simulink subsystem "Regler"  (R2021b)
settings: Solver=VariableStepAuto  StartTime=0.0  StopTime=10.0  RelTol=1e-3
undefined symbols (not defined in the file or in its folder): SimParam
settings Model: Creator=tim  LastModifiedBy=tim

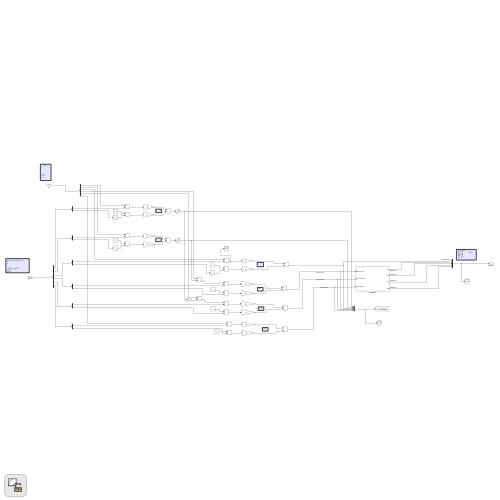
[thumbnail: Simulink's stored preview of the top-level diagram]
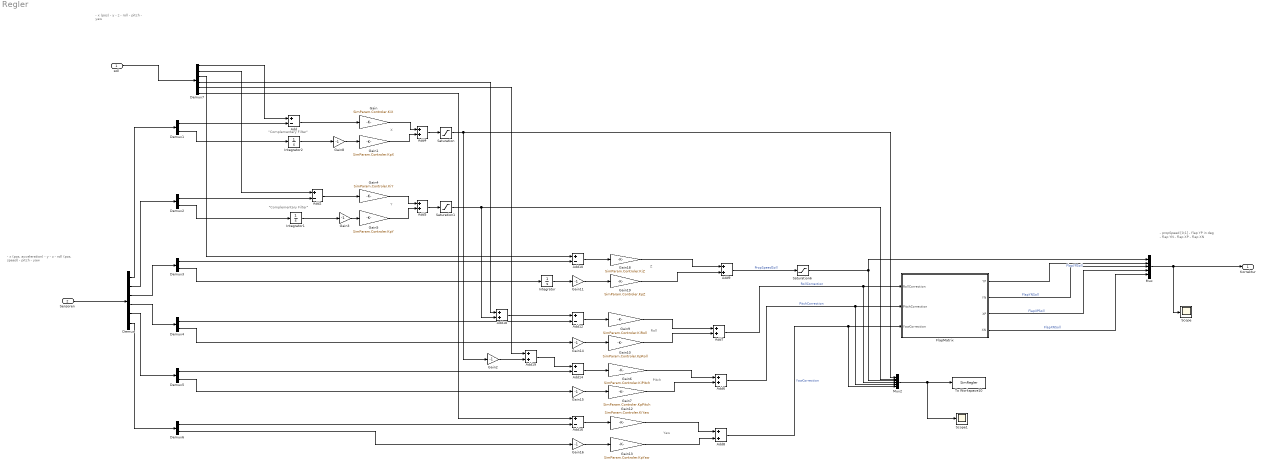
== system Regler ==
  note: Z
  note: - x (pos, acceleration)
      | - y
      | - z
      |
      |
      | - roll (pos, speed)
      | - pitch
      | - yaw
  note: Y
  note: X
  note: Pitch
  note: Roll
  note: Yaw
  note: - propSpeed [0;1]
      | - flap YP          in deg
      | - flap YN
      | - flap XP
      | - flap XN
  note: - x (pos)
      | - y
      | - z
      |
      |
      | - roll
      | - pitch
      | - yaw
  note: "Complementary Filter"
  note: "Complementary Filter"
  soll : Inport
  Sensoren : Inport  Port=2
  Add{,2,10,12,14,16} (6 alike) : Sum  Inputs=+-
  Add{4..9,18..19} (8 alike) : Sum
  Demux : Demux  Outputs=6
  Demux{1..6} (6 alike) : Demux  Outputs=2
  Demux7 : Demux  Outputs=6
  FlapMatrix : Subsystem
  Gain : Gain  Gain=SimParam.Controler.KiX
  Gain1 : Gain  Gain=SimParam.Controler.KpX
  Gain10 : Gain  Gain=SimParam.Controler.KpRoll
  Gain{2..3,8,11,14..16} (7 alike) : Gain  Gain=-1
  Gain12 : Gain  Gain=SimParam.Controler.KiYaw
  Gain13 : Gain  Gain=SimParam.Controler.KpYaw
  Gain18 : Gain  Gain=SimParam.Controler.KiZ
  Gain19 : Gain  Gain=SimParam.Controler.KpZ
  Gain4 : Gain  Gain=SimParam.Controler.KiY
  Gain5 : Gain  Gain=SimParam.Controler.KpY
  Gain6 : Gain  Gain=SimParam.Controler.KiPitch
  Gain7 : Gain  Gain=SimParam.Controler.KpPitch
  Gain9 : Gain  Gain=SimParam.Controler.KiRoll
  Integrator : Integrator
  Integrator1 : Integrator
  Integrator2 : Integrator
  Mux : Mux  Inputs=5
  Mux2 : Mux  Inputs=6
  Saturation : Saturate  UpperLimit=SimParam.Physics.MaxTiltActuation  LowerLimit=-SimParam.Physics.MaxTiltActuation
  Saturation1 : Saturate  UpperLimit=SimParam.Physics.MaxTiltActuation  LowerLimit=-SimParam.Physics.MaxTiltActuation
  Saturation6 : Saturate  UpperLimit=0  LowerLimit=-1
  Scope : Scope
  Scope1 : Scope
  To Workspace10 : ToWorkspace  VariableName=SimRegler  SaveFormat=Timeseries  SampleTime=-1
  Korrektur : Outport
  wires:
  soll/1 -> Demux7/1
  Mux/1 -> Korrektur/1, Scope/1
  Add9/1 -> Saturation6/1  "PropSpeedSoll"
  Add4/1 -> Saturation/1
  Add5/1 -> Saturation1/1
  Add7/1 -> FlapMatrix/1(RollCorrection), Mux2/4  "RollCorrection"
  FlapMatrix/4(XN) -> Mux/5  "FlapXNSoll"
  FlapMatrix/3(XP) -> Mux/4  "FlapXPSoll"
  FlapMatrix/2(YN) -> Mux/3  "FlapYNSoll"
  FlapMatrix/1(YP) -> Mux/2  "FlapYPSoll"
  Add6/1 -> FlapMatrix/2(PitchCorrection), Mux2/5  "PitchCorrection"
  Gain4/1 -> Add5/1
  Gain5/1 -> Add5/2
  Gain6/1 -> Add6/1
  Gain7/1 -> Add6/2
  Gain9/1 -> Add7/1
  Gain10/1 -> Add7/2
  Add8/1 -> FlapMatrix/3(YawCorrection), Mux2/6  "YawCorrection"
  Gain12/1 -> Add8/1
  Gain13/1 -> Add8/2
  Gain18/1 -> Add9/1
  Gain19/1 -> Add9/2
  Mux2/1 -> To Workspace10/1, Scope1/1
  Sensoren/1 -> Demux/1
  Demux/6 -> Demux6/1
  Demux/5 -> Demux5/1
  Demux/4 -> Demux4/1
  Demux/3 -> Demux3/1
  Demux/2 -> Demux2/1
  Demux/1 -> Demux1/1
  Add/1 -> Gain/1
  Integrator2/1 -> Gain8/1
  Add2/1 -> Gain4/1
  Gain3/1 -> Gain5/1
  Add10/1 -> Gain18/1
  Integrator/1 -> Gain11/1
  Add12/1 -> Gain9/1
  Add14/1 -> Gain6/1
  Gain15/1 -> Gain7/1
  Add16/1 -> Gain12/1
  Demux6/2 -> Gain16/1
  Demux7/1 -> Add/1
  Demux7/2 -> Add2/1
  Demux7/3 -> Add10/1
  Demux7/4 -> Add18/1
  Demux7/5 -> Add19/1
  Demux7/6 -> Add16/1
  Add19/1 -> Add14/1
  Add18/1 -> Add12/1
  Demux1/1 -> Add/2
  Demux1/2 -> Integrator2/1
  Demux2/1 -> Add2/2
  Demux2/2 -> Integrator1/1
  Demux3/1 -> Add10/2
  Demux3/2 -> Integrator/1
  Demux4/1 -> Add12/2
  Demux5/1 -> Add14/2
  Demux5/2 -> Gain15/1
  Demux6/1 -> Add16/2
  Integrator1/1 -> Gain3/1
  Gain/1 -> Add4/1
  Gain1/1 -> Add4/2
  Gain2/1 -> Add19/2
  Saturation/1 -> Mux2/1, Gain2/1
  Saturation1/1 -> Add18/2, Mux2/2
  Gain8/1 -> Gain1/1
  Gain11/1 -> Gain19/1
  Gain14/1 -> Gain10/1
  Demux4/2 -> Gain14/1
  Gain16/1 -> Gain13/1
  Saturation6/1 -> Mux2/3, Mux/1

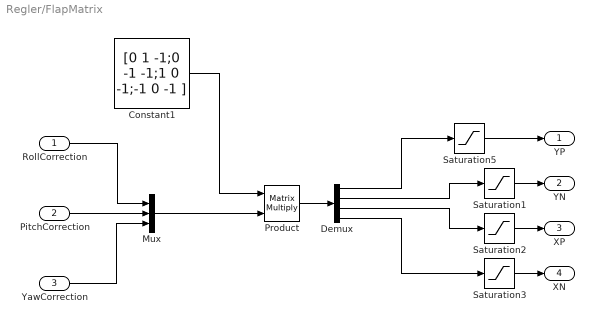
== system Regler/FlapMatrix ==
  RollCorrection : Inport
  PitchCorrection : Inport  Port=2
  YawCorrection : Inport  Port=3
  Constant1 : Constant  Value=[0 1 -1;0 -1 -1;1 0 -1;-1 0 -1 ]
  Demux : Demux
  Mux : Mux  Inputs=3
  Product : Product  Multiplication=Matrix(*)
  Saturation{1..3,5} (4 alike) : Saturate  UpperLimit=SimParam.Physics.MaxFlapAngle  LowerLimit=-SimParam.Physics.MaxFlapAngle
  YP : Outport
  YN : Outport  Port=2
  XP : Outport  Port=3
  XN : Outport  Port=4
  wires:
  Saturation3/1 -> XN/1
  Saturation2/1 -> XP/1
  Saturation1/1 -> YN/1
  Saturation5/1 -> YP/1
  Demux/4 -> Saturation3/1
  Demux/3 -> Saturation2/1
  Demux/2 -> Saturation1/1
  Demux/1 -> Saturation5/1
  Product/1 -> Demux/1
  Constant1/1 -> Product/1
  Mux/1 -> Product/2
  YawCorrection/1 -> Mux/3
  PitchCorrection/1 -> Mux/2
  RollCorrection/1 -> Mux/1
